simulink model "gfc199A_yen"  (Simulink 8.5)
settings: Solver=ode45  StartTime=0.0  StopTime=10  FixedStep=Ts  RelTol=1e-3
values from neighbouring files (symbols this model uses):
  K = 32    [main.m]
  Nce = 2    [main.m]
  Ne = 1    [main.m]
  Nu = 3    [main.m]
  Ts = 0.5    [main.m]
libraries: fuzblock x1
settings Model: Creator=Steve  LastModifiedBy=user  ExtModeTrigMode=oneshot  ExtModeArmWhenConnect=off
settings DataIOCC: LimitDataPoints=off  SaveOutput=off  SignalLogging=off  DSMLogging=off  VisualizeSimOutput=off  SaveTime=off
settings OptimizationCC: BlockReduction=off  BooleanDataType=off  InitFltsAndDblsToZero=on
settings DebuggingCC: SaveWithParameterizedLinksMsg=none  SignalResolutionControl=TryResolveAllWithWarning  MultiTaskDSMMsg=warning  MultiTaskCondExecSysMsg=none  FcnCallInpInsideContextMsg=UseLocalSettings
settings HardwareCC: TargetUnknown=on

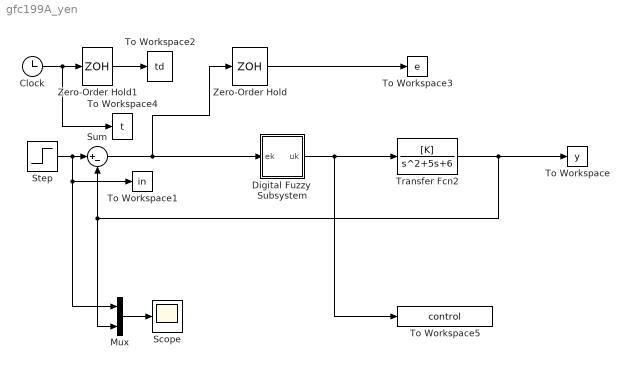
== system gfc199A_yen ==
  Clock : Clock
  Digital Fuzzy  Subsystem : Subsystem
  Mux : Mux  Inputs=2
  Scope : Scope
      settings: TimeRange=20  YMax=15  MaxDataPoints=50000
  Step : Step  Time=0  SampleTime=0
  Sum : Sum  Inputs=|+-  SaturateOnIntegerOverflow=on  InputSameDT=on  OutDataTypeStr=Inherit: Same as first input
  To Workspace : ToWorkspace  VariableName=y  SampleTime=-1
  To Workspace1 : ToWorkspace  VariableName=in  SampleTime=-1
  To Workspace2 : ToWorkspace  VariableName=td  SampleTime=-1
  To Workspace3 : ToWorkspace  VariableName=e  SampleTime=-1
  To Workspace4 : ToWorkspace  VariableName=t  SampleTime=-1
  To Workspace5 : ToWorkspace  VariableName=control  SampleTime=-1
  Transfer Fcn2 : TransferFcn  Numerator=[K]  Denominator=[1 5 6]
  Zero-Order Hold : ZeroOrderHold  SampleTime=Ts
  Zero-Order Hold1 : ZeroOrderHold  SampleTime=Ts
  wires:
  Digital Fuzzy  Subsystem/1(uk) -> To Workspace5/1, Transfer Fcn2/1
  Transfer Fcn2/1 -> To Workspace/1, Sum/2, Mux/2
  Step/1 -> Sum/1, To Workspace1/1, Mux/1
  Clock/1 -> To Workspace4/1, Zero-Order Hold1/1
  Sum/1 -> Digital Fuzzy  Subsystem/1(ek), Zero-Order Hold/1
  Mux/1 -> Scope/1
  Zero-Order Hold/1 -> To Workspace3/1
  Zero-Order Hold1/1 -> To Workspace2/1

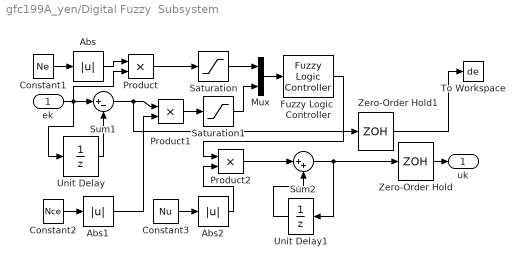
== system gfc199A_yen/Digital Fuzzy  Subsystem ==
  ek : Inport
  Abs : Abs  SaturateOnIntegerOverflow=on
  Abs1 : Abs  SaturateOnIntegerOverflow=on
  Abs2 : Abs  SaturateOnIntegerOverflow=on
  Constant1 : Constant  Value=Ne
  Constant2 : Constant  Value=Nce
  Constant3 : Constant  Value=Nu
  Fuzzy Logic  Controller : fuzblock/Fuzzy Logic  Controller  fis=gfc
  Mux : Mux  Inputs=2
  Product : Product  SaturateOnIntegerOverflow=on  RndMeth=Zero  InputSameDT=on  OutDataTypeStr=Inherit: Same as first input
  Product1 : Product  SaturateOnIntegerOverflow=on  RndMeth=Zero  InputSameDT=on  OutDataTypeStr=Inherit: Same as first input
  Product2 : Product  SaturateOnIntegerOverflow=on  RndMeth=Zero  InputSameDT=on  OutDataTypeStr=Inherit: Same as first input
  Saturation : Saturate  UpperLimit=1  LowerLimit=-1
  Saturation1 : Saturate  UpperLimit=1  LowerLimit=-1
  Sum1 : Sum  Inputs=|+-  SaturateOnIntegerOverflow=on  InputSameDT=on  OutDataTypeStr=Inherit: Same as first input
  Sum2 : Sum  Inputs=|++  SaturateOnIntegerOverflow=on  InputSameDT=on  OutDataTypeStr=Inherit: Same as first input
  To Workspace : ToWorkspace  VariableName=de  SampleTime=-1
  Unit Delay : UnitDelay  SampleTime=Ts
  Unit Delay1 : UnitDelay  SampleTime=Ts
  Zero-Order Hold : ZeroOrderHold  SampleTime=Ts
  Zero-Order Hold1 : ZeroOrderHold  SampleTime=Ts
  uk : Outport
  wires:
  ek/1 -> Sum1/1, Unit Delay/1, Product/2
  Unit Delay/1 -> Sum1/2
  Sum1/1 -> Product1/1, Zero-Order Hold1/1
  Product1/1 -> Saturation1/1
  Product/1 -> Saturation/1
  Mux/1 -> Fuzzy Logic  Controller/1
  Fuzzy Logic  Controller/1 -> Product2/1
  Zero-Order Hold/1 -> uk/1
  Unit Delay1/1 -> Sum2/2
  Sum2/1 -> Unit Delay1/1, Zero-Order Hold/1
  Abs/1 -> Product/1
  Constant1/1 -> Abs/1
  Constant2/1 -> Abs1/1
  Abs1/1 -> Product1/2
  Product2/1 -> Sum2/1
  Constant3/1 -> Abs2/1
  Abs2/1 -> Product2/2
  Zero-Order Hold1/1 -> To Workspace/1
  Saturation/1 -> Mux/1
  Saturation1/1 -> Mux/2
